simulink model "V126_L7_UMS"  (R2020b)
settings: Solver=VariableStepAuto  StartTime=0.0  StopTime=100  MaxStep=0.01  RelTol=1e-3
undefined symbols (not defined in the file): Cd, F, K, K1, K2, Kg, m0, m1, m2, q, T1, T2, T3, Ts, Un
settings Model: Creator=td  LastModifiedBy=Maxim
settings DataIOCC: ReturnWorkspaceOutputs=off
settings DebuggingCC: ArithmeticOperatorsInVariantConditions=warning
settings SFSimCC: CustomCodeUndefinedFunction=UseInterfaceOnly

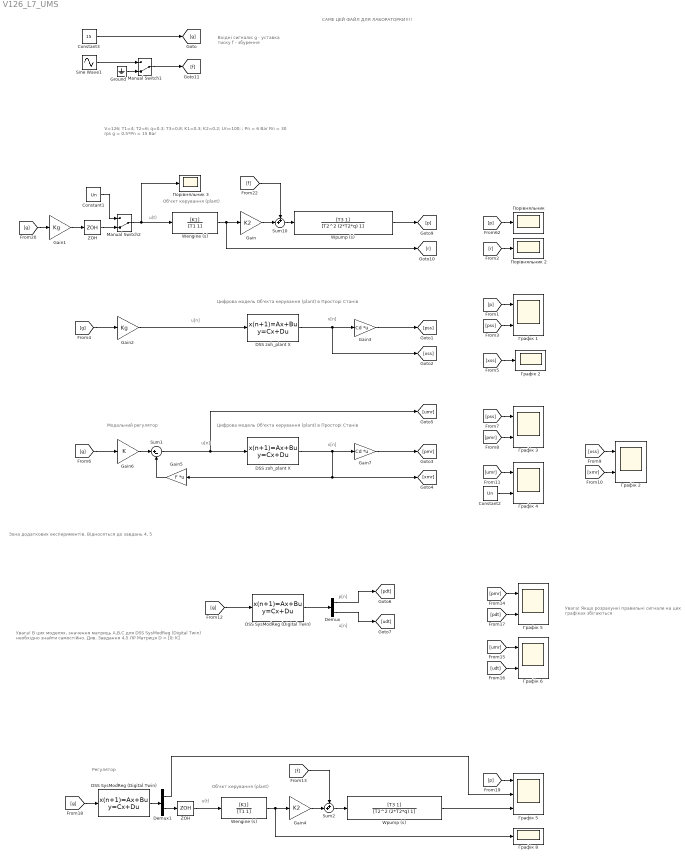
== system V126_L7_UMS ==
  note: Увага!
      | В цих моделях, значення матриць A,B,C для DSS SysModReg (Digital Twin) необхідно знайти самостійно. Див. Завдання 4,5 ЛР
      | Матриця D = [0; K]
  note: Зона додаткових експериментів. Відносяться до завдань 4, 5
  note: Регулятор
  note: Модальний регулятор
  note: x[n]
  note: u(t)
  note: V=126; T1=4; T2=6; q=0.3; T3=0.8; K1=0.3; K2=0.2; Un=100; ;
      |
      | Pn = 6 Bar
      | Rn = 30 rps
      |
      | g = 0.5*Pn = 15 Bar
  note: Вхідні сигнали:
      |
      | g - уставка тиску
      |
      | f - збурення
  note: САМЕ ЦЕЙ ФАЙЛ
      | ДЛЯ ЛАБОРАТОРКИ!!!!
  note: Об'єкт керування (plant)
  note: Цифрова модель Об'єкта керування (plant) в Просторі Станів
  note: u[n]
  note: Цифрова модель Об'єкта керування (plant) в Просторі Станів
  note: u[n]
  note: x[n]
  note: u(t)
  note: Об'єкт керування (plant)
  note: u[n]
  note: p[n]
  note: Увага!
      | Якщо розрахункі правильні
      | сигнали на цих графіках збігаються
  "  Wpump (s)" : TransferFcn  Numerator=[T3 1]  Denominator=[T2^2 (2*T2*q) 1]
  "  Wpump (s) " : TransferFcn  Numerator=[T3 1]  Denominator=[T2^2 (2*T2*q) 1]
  " DSS SysModReg (Digital Twin)" : DiscreteStateSpace  A=0  B=0  C=[0; 0]  D=[0; K]  SampleTime=Ts
  " DSS SysModReg (Digital Twin) " : DiscreteStateSpace  A=0  B=0  C=[0; 0]  D=[0; K]  SampleTime=Ts
  " DSS zoh_plant X" : DiscreteStateSpace  A="[ 0 1 0 ; 0 0 1 ;  -m0  -m1  -m2 ]"  B=[ 0 ; 0 ; 1 ]  C=eye(3)  D=[0;0;0]  SampleTime=Ts
  " DSS zoh_plant X " : DiscreteStateSpace  A="[ 0 1 0 ; 0 0 1 ;  -m0  -m1  -m2 ]"  B=[ 0 ; 0 ; 1 ]  C=[1 0 0; 0 1 0; 0 0 1]  D=[0;0;0]  SampleTime=Ts
  " ZOH " : ZeroOrderHold  SampleTime=Ts
  " Графік 2" : Scope
  " Графік 5  " : Scope  NumInputPorts=3
  " Порівняльник " : Scope
  " Порівняльник 2" : Scope
  " Порівняльник 3" : Scope
  Constant1 : Constant  Value=Un
  Constant2 : Constant  Value=Un
  Constant3 : Constant  Value=15
  Demux : Demux  Outputs=2
  Demux1 : Demux  Outputs=2
  Gain : Gain  Gain=K2
  Gain1 : Gain  Gain=Kg
  Gain2 : Gain  Gain=Kg
  Gain3 : Gain  Gain=Cd  Multiplication=Matrix(K*u)
  Gain4 : Gain  Gain=K2
  Gain5 : Gain  Gain=F  Multiplication=Matrix(K*u)
  Gain6 : Gain  Gain=K
  Gain7 : Gain  Gain=Cd  Multiplication=Matrix(K*u)
  Ground : Ground
  Manual Switch1 : ManualSwitch  CurrentSetting=0
  Manual Switch2 : ManualSwitch  CurrentSetting=0
  Sine Wave1 : Sin  Amplitude=5  Frequency=0.4  SampleTime=Ts
  Sum1 : Sum  Inputs=|+-
  Sum10 : Sum  Inputs=++|
  Sum2 : Sum  Inputs=++|
  "Wengine (s) " : TransferFcn  Numerator=[K1]  Denominator=[T1 1]
  "Wengine (s)  " : TransferFcn  Numerator=[K1]  Denominator=[T1 1]
  ZOH : ZeroOrderHold  SampleTime=Ts
  Графік {1..6} (6 alike) : Scope  NumInputPorts=2
  Графік 8 : Scope
  wires:
  Sine Wave1/1 -> Manual Switch1/1
  Gain/1 -> Sum10/2
  Sum10/1 -> "  Wpump (s)"/1
  Manual Switch1/1 -> [f]
  "  Wpump (s)"/1 -> [p]
  [f] -> Sum10/1
  Constant3/1 -> [g]
  "Wengine (s) "/1 -> Gain/1, [r]
  [p] -> " Порівняльник "/1
  Manual Switch2/1 -> "Wengine (s) "/1, " Порівняльник 3"/1
  ZOH/1 -> Manual Switch2/2
  Constant1/1 -> Manual Switch2/1
  Ground/1 -> Manual Switch1/2
  [r] -> " Порівняльник 2"/1
  Gain1/1 -> ZOH/1
  [g] -> Gain1/1
  Gain2/1 -> " DSS zoh_plant X "/1
  " DSS zoh_plant X "/1 -> [xss], Gain3/1
  Gain3/1 -> [pss]
  [p] -> Графік 1/1
  [pss] -> Графік 1/2
  [g] -> Gain2/1
  [xss] -> " Графік 2"/1
  " DSS zoh_plant X"/1 -> Gain5/1, [xmr], Gain7/1
  Gain7/1 -> [pmr]
  [g] -> Gain6/1
  Gain6/1 -> Sum1/1
  Sum1/1 -> [umr], " DSS zoh_plant X"/1
  Gain5/1 -> Sum1/2
  [pmr] -> Графік 3/2
  [pss] -> Графік 3/1
  [xss] -> Графік 2/1
  [xmr] -> Графік 2/2
  [umr] -> Графік 4/1
  Constant2/1 -> Графік 4/2
  [g] -> " DSS SysModReg (Digital Twin)"/1
  " DSS SysModReg (Digital Twin)"/1 -> Demux/1
  Demux/1 -> [pdt]
  Demux/2 -> [udt]
  [umr] -> Графік 6/1
  [udt] -> Графік 6/2
  [pdt] -> Графік 5/2
  [pmr] -> Графік 5/1
  "Wengine (s)  "/1 -> Графік 8/1, Gain4/1
  [f] -> Sum2/1
  Gain4/1 -> Sum2/2
  Sum2/1 -> "  Wpump (s) "/1
  [g] -> " DSS SysModReg (Digital Twin) "/1
  " DSS SysModReg (Digital Twin) "/1 -> Demux1/1
  Demux1/2 -> " ZOH "/1
  " ZOH "/1 -> "Wengine (s)  "/1
  [p] -> " Графік 5  "/1
  "  Wpump (s) "/1 -> " Графік 5  "/3
  Demux1/1 -> " Графік 5  "/2
